simulink model "Lab1Test"  (R2021a)
settings: Solver=FixedStepAuto  StartTime=0.0  StopTime=0.15  FixedStep=1e-5  RelTol=1e-3
values from neighbouring files (symbols this model uses):
  d = 0.6    [Lab1Exp1.m]    (also in Lab1Teste2.m)
  ILi = 0    [Lab1Teste2.m]
  K1 = 1/L    (= 1000)    [CC.m]    (also in Lab1Teste2.m)
  K2 = -K1*rl    (= 0)    [CC.m]    (also in Lab1Teste2.m)
  K3 = 1/C    (= 454.545454545)    [CC.m]    (also in Lab1Teste2.m)
  K4 = -K3/R    (= -113.636363636)    [CC.m]    (also in Lab1Teste2.m)
  Po = 10    [CC.m]    (also in Conversor.m; Lab1Exp1.m = PoV(k); Lab1Teste2.m)
  To = 0.08    [Lab1Teste2.m]
  u0 = 0.05    [Lab1Exp1.m]    (also in Lab1Teste2.m = 0)
  Vci = 1e-1    (= 0.1)    [Lab1Teste2.m]
  Vin = 20    [CC.m]    (also in Conversor.m; Lab1Exp1.m; Lab1Teste2.m)
settings Model: Creator=DaniSan  LastModifiedBy=DaniSan

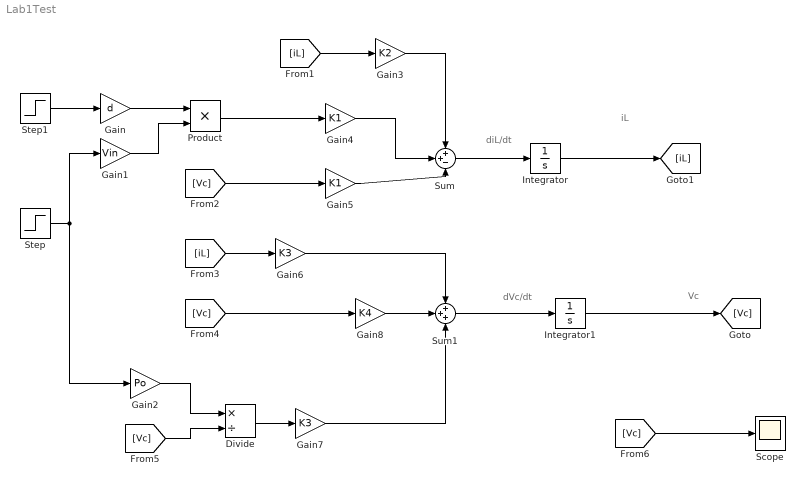
== system Lab1Test ==
  note: iL
  note: diL/dt
  note: dVc/dt
  note: Vc
  Divide : Product  Inputs=*/
  Gain : Gain  Gain=d
  Gain1 : Gain  Gain=Vin
  Gain2 : Gain  Gain=Po
  Gain3 : Gain  Gain=K2
  Gain4 : Gain  Gain=K1
  Gain5 : Gain  Gain=K1
  Gain6 : Gain  Gain=K3
  Gain7 : Gain  Gain=K3
  Gain8 : Gain  Gain=K4
  Integrator : Integrator  InitialCondition=ILi
  Integrator1 : Integrator  InitialCondition=Vci  UpperSaturationLimit=Vin
  Product : Product
  Scope : Scope
  Step : Step  Time=0  SampleTime=0
  Step1 : Step  Time=To  Before=1  After=1+u0/d  SampleTime=0
  Sum : Sum  Inputs=++-
  Sum1 : Sum  Inputs=+++
  wires:
  Step/1 -> Gain1/1, Gain2/1
  Gain/1 -> Product/1
  Product/1 -> Gain4/1
  Gain4/1 -> Sum/2
  Sum/1 -> Integrator/1
  Gain3/1 -> Sum/1
  Sum1/1 -> Integrator1/1
  Gain5/1 -> Sum/3
  Gain6/1 -> Sum1/1
  Divide/1 -> Gain7/1
  Gain7/1 -> Sum1/3
  Gain8/1 -> Sum1/2
  Integrator/1 -> [iL]
  [iL] -> Gain3/1
  [Vc] -> Gain5/1
  [iL] -> Gain6/1
  [Vc] -> Gain8/1
  [Vc] -> Divide/2
  [Vc] -> Scope/1
  Gain2/1 -> Divide/1
  Gain1/1 -> Product/2
  Integrator1/1 -> [Vc]
  Step1/1 -> Gain/1
